simulink model "SumaSTenSimulink"  (R2015a)
settings: Solver=ode45  StartTime=0.0  StopTime=1E-12  RelTol=1e-3
libraries: simulink x6
settings Model: Creator=MEGAS PC  LastModifiedBy=MEGAS PC

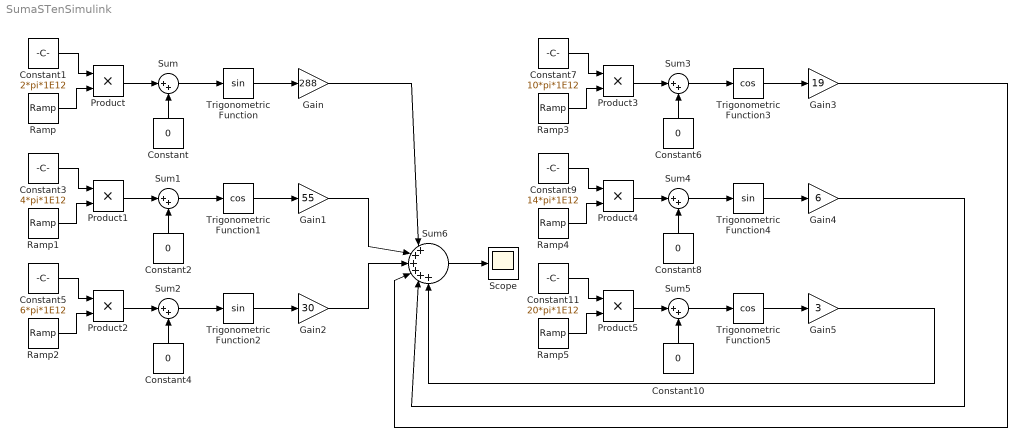
== system SumaSTenSimulink ==
  Constant{,2,4,6,8,10} (6 alike) : Constant  Value=0
  Constant1 : Constant  Value=2*pi*1E12
  Constant11 : Constant  Value=20*pi*1E12
  Constant3 : Constant  Value=4*pi*1E12
  Constant5 : Constant  Value=6*pi*1E12
  Constant7 : Constant  Value=10*pi*1E12
  Constant9 : Constant  Value=14*pi*1E12
  Gain : Gain  Gain=288
  Gain1 : Gain  Gain=55
  Gain2 : Gain  Gain=30
  Gain3 : Gain  Gain=19
  Gain4 : Gain  Gain=6
  Gain5 : Gain  Gain=3
  Product{,1..5} (6 alike) : Product
  Ramp{,1..5} (6 alike) : simulink/Sources/Ramp  slope=1  start=0  X0=1E-15
  Scope : Scope
      settings: YMin=78.5  YMax=81
  Sum{,1..5} (6 alike) : Sum  Inputs=|++
  Sum6 : Sum  Inputs=|++++++
  Trigonometric Function : Trigonometry
  Trigonometric Function1 : Trigonometry  Operator=cos
  Trigonometric Function2 : Trigonometry
  Trigonometric Function3 : Trigonometry  Operator=cos
  Trigonometric Function4 : Trigonometry
  Trigonometric Function5 : Trigonometry  Operator=cos
  wires:
  Constant1/1 -> Product/1
  Product/1 -> Sum/1
  Constant/1 -> Sum/2
  Sum/1 -> Trigonometric Function/1
  Trigonometric Function/1 -> Gain/1
  Ramp/1 -> Product/2
  Constant3/1 -> Product1/1
  Product1/1 -> Sum1/1
  Constant2/1 -> Sum1/2
  Sum1/1 -> Trigonometric Function1/1
  Trigonometric Function1/1 -> Gain1/1
  Ramp1/1 -> Product1/2
  Constant5/1 -> Product2/1
  Product2/1 -> Sum2/1
  Constant4/1 -> Sum2/2
  Sum2/1 -> Trigonometric Function2/1
  Trigonometric Function2/1 -> Gain2/1
  Ramp2/1 -> Product2/2
  Constant7/1 -> Product3/1
  Product3/1 -> Sum3/1
  Constant6/1 -> Sum3/2
  Sum3/1 -> Trigonometric Function3/1
  Trigonometric Function3/1 -> Gain3/1
  Ramp3/1 -> Product3/2
  Constant9/1 -> Product4/1
  Product4/1 -> Sum4/1
  Constant8/1 -> Sum4/2
  Sum4/1 -> Trigonometric Function4/1
  Trigonometric Function4/1 -> Gain4/1
  Ramp4/1 -> Product4/2
  Constant11/1 -> Product5/1
  Product5/1 -> Sum5/1
  Constant10/1 -> Sum5/2
  Sum5/1 -> Trigonometric Function5/1
  Trigonometric Function5/1 -> Gain5/1
  Ramp5/1 -> Product5/2
  Gain/1 -> Sum6/1
  Gain2/1 -> Sum6/3
  Gain3/1 -> Sum6/4
  Gain5/1 -> Sum6/6
  Gain4/1 -> Sum6/5
  Sum6/1 -> Scope/1
  Gain1/1 -> Sum6/2
